simulink model "Step_6"  (R2024b)
settings: Solver=VariableStepAuto  StartTime=0.0  StopTime=1000.0  RelTol=1e-3
libraries: dspsrcs4 x1
settings Model: Creator=Omar  LastModifiedBy=Omar

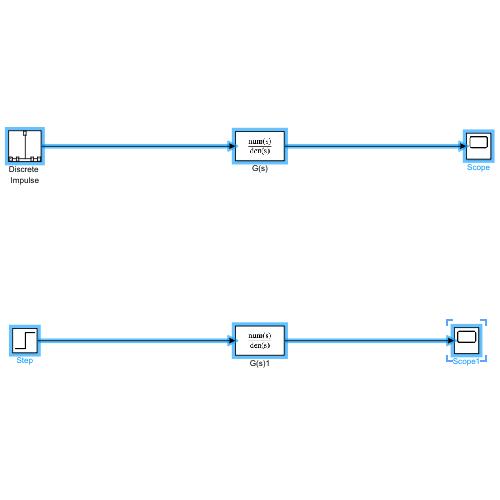
[thumbnail: Simulink's stored preview of the top-level diagram]
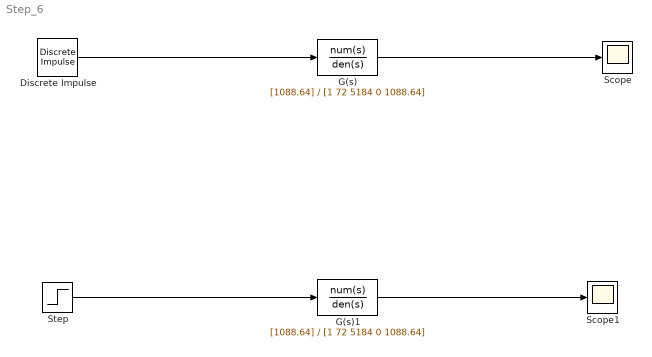
== system Step_6 ==
  Discrete Impulse : dspsrcs4/Discrete  Impulse  Delay=0  SampleTime=1  FrameSample=1  OutputFrames=off  dataType=double  isSigned=on  wordLen=16  udDataType=sfix(16)  fracBitsMode=Best precision  numFracBits=15  OutDataTypeStr=double  LastOutDataTypeStr=double
  G(s) : TransferFcn  Numerator=[1088.64]  Denominator=[1 72 5184 0 1088.64]
  G(s)1 : TransferFcn  Numerator=[1088.64]  Denominator=[1 72 5184 0 1088.64]
  Scope : Scope
  Scope1 : Scope
  Step : Step  SampleTime=0
  wires:
  G(s)1/1 -> Scope1/1
  Discrete Impulse/1 -> G(s)/1
  G(s)/1 -> Scope/1
  Step/1 -> G(s)1/1
